simulink model "zad1Model"  (R2012b)
settings: Solver=ode45  StartTime=0.0  StopTime=10.0  MaxStep=0.198  RelTol=1e-3
settings Model: Creator=VolAnder  LastModifiedBy=VoAnder

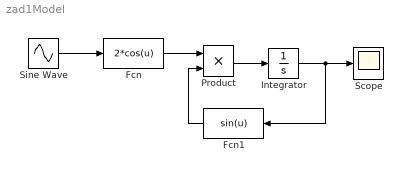
== system zad1Model ==
  Fcn : Fcn  Expr=2*cos(u)
  Fcn1 : Fcn  Expr=sin(u)
  Integrator : Integrator  InitialCondition=0.1
  Product : Product  RndMeth=Zero
  Scope : Scope
  Sine Wave : Sin  SampleTime=0
  wires:
  Sine Wave/1 -> Fcn/1
  Fcn/1 -> Product/1
  Product/1 -> Integrator/1
  Integrator/1 -> Fcn1/1, Scope/1
  Fcn1/1 -> Product/2
